simulink model "Drive_Cycle_Sim"  (R2020a)
settings: Solver=FixedStepAuto  StartTime=0  StopTime=108.92  FixedStep=0.01  MinStep=0.001  RelTol=1e-3
undefined symbols (not defined in the file or in its folder): Accumulator, Brakes, Driver, Gearbox, k_coulombToampHour, k_joulesTokWH, Motor, PedalMap, Regen, SimVehicle, Speed, Tire
libraries: autolibshared x3, simulink x2, dspstat3 x1
settings Model: Creator=Harjot  LastModifiedBy=harjo

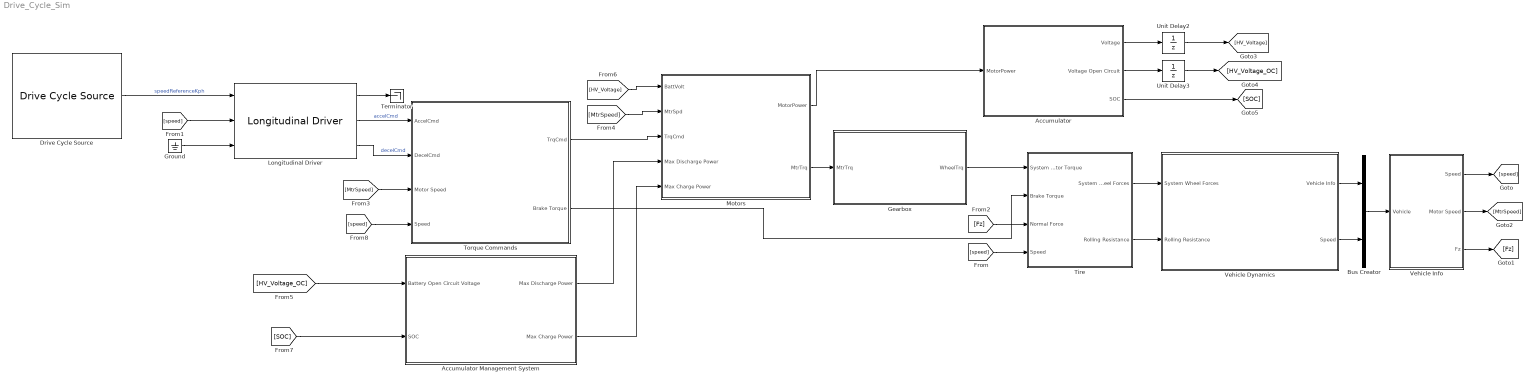
== system Drive_Cycle_Sim ==
  Accumulator : Subsystem
      mask Display: image('C:\Users\harjo\Downloads\battery.png'); % Use "Edit Image" on toolstrip to change.
  Accumulator Management System : Subsystem
      mask Display: image('C:\Users\harjo\Downloads\ams.jpg'); % Use "Edit Image" on toolstrip to change.
  Bus Creator : BusCreator  Inputs=2
  Drive Cycle Source : autolibshared/Drive Cycle Source  cycleVar=Workspace variable  wsVar=drivecycle  fileVar=cycleFTP75.mat  tfinal="108.92  seconds, Cyclic"  cycleRepeat=on  outAccPort=off  outGearPort=off  gearList=No gear data  t_wot1=5  xdot_woto=0  xdot_wot1=30  t_wot2=20  xdot_wot2=0  t_wotend=30  srcUnit=km/h  outUnit=km/hr  srcAccUnit=m/s/s  outAccUnit=m/s^2  dt=0.01  aMode=2  faultOption=off  velBnd=2  velBndUnit=mph  inUnit=m/s  timeBnd=1  failOption=off  stopSim=off  maxFaultCnt=10  maxFaultTime=2  maxTotFaultTime=15  traceOption=off  dtTrace=1  traceWindow=10  lastDCname=Custom Data Set  lastOutUnit=mph  lastDT=0.01  lastTB=1  lastSB=2  forceCalcBound=off
      settings: SourceProductBaseCode=PW,MT,VE,VP
  Gearbox : Subsystem
      mask Display: image('C:\Users\harjo\Downloads\gearbox.png'); % Use "Edit Image" on toolstrip to change.
  Ground : Ground
  Longitudinal Driver : autolibshared/Longitudinal Driver  extAccelOvr=off  extDecelOvr=off  extAccelHld=off  extDecelHld=off  extAccelZero=off  extDecelZero=off  cntrlType=PI  shftType=None  velUnits=km/hr  gearOut=off  Kp=Driver.k_kp  Ki=Driver.k_ki  Kff=Driver.k_kff  Kg=Driver.k_kg  VehVelVec=[0 100]  KffVec=[.1 .1]  KpVec=[10 10]  KiVec=[5 5]  KgVec=[0 0]  m=1500  Kpt=3000  tau=.1  L=2  aR=200  bR=2.5  cR=.5  g=9.81  vnom=Driver.k_vnom  Kaw=Driver.k_kaw  tauerr=Driver.k_tauerr  tauPt=2  GearInit=0  tShift=.1  pdlVec=[0.1 0.4 0.5 0.9]  upShftTbl=[-1 12.9375 26.4375 39.9375 51.18749999999999 62.4375 72.84375 83.25;-1 16.3125 29.8125 43.3125 54.5624 65.8125 76.78125 87.75;-1 19.6875 33.1875 46.68749999999999 57.9375 69.1875 80.71875 92.25;-1 33 52.5 77.25 100.5 138.75 161.875 185]  dwnShftTbl=[1 9.5625 23.0625 36.5625 47.8125 59.0625 68.90625 78.75;1 12.9375 26.4375 39.9375 51.18749999999999 62.4375 72.84375 83.25;1 16.3125 29.8125 43.3125 54.562499 65.8125 76.78125 87.75;1 19.6875 33.1875 46.68749999999999 57.9375 69.1875 80.71875 92.25]  tClutch=.5  tRev=.5  tPark=120  aMode=1  UpGearVec="[0  1  2  3  4  5  6  7]"  DownGearVec="[1  2  3  4  5  6  7  8]"
      settings: SourceProductBaseCode=PW,MT,VE,VP
  Motors : Subsystem
      mask Display: image('C:\Users\harjo\Downloads\motor.png'); % Use "Edit Image" on toolstrip to change.
  Terminator : Terminator
  Tire : Subsystem
      mask Display: image('C:\Users\harjo\Downloads\tire.jpg'); % Use "Edit Image" on toolstrip to change.
  Torque Commands : Subsystem
  Unit Delay2 : UnitDelay  InitialCondition=Accumulator.k_initialPackVoltage  SampleTime=-1  HasFrameUpgradeWarning=on
  Unit Delay3 : UnitDelay  InitialCondition=Accumulator.k_maxCellVoltage  SampleTime=-1  HasFrameUpgradeWarning=on
  Vehicle Dynamics : Subsystem
      mask Display: image('C:\Users\harjo\Downloads\carZapdos.png'); % Use "Edit Image" on toolstrip to change.
  Vehicle Info : Subsystem
  wires:
  Gearbox/1(WheelTrq) -> Tire/1(System Motor Torque)
  [MtrSpeed] -> Torque Commands/3(Motor Speed)
  Torque Commands/2(Brake Torque) -> Tire/2(Brake Torque)
  Tire/2(Rolling Resistance) -> Vehicle Dynamics/2(Rolling Resistance)
  Tire/1(System Wheel Forces) -> Vehicle Dynamics/1(System Wheel Forces)
  Drive Cycle Source/1 -> Longitudinal Driver/1  "speedReferenceKph"
  [Fz] -> Tire/3(Normal Force)
  [speed] -> Tire/4(Speed)
  Unit Delay2/1 -> [HV_Voltage]
  Accumulator/1(Voltage) -> Unit Delay2/1
  [HV_Voltage] -> Motors/1(BattVolt)
  Accumulator/2(Voltage Open Circuit) -> Unit Delay3/1
  Unit Delay3/1 -> [HV_Voltage_OC]
  [MtrSpeed] -> Motors/2(MtrSpd)
  Motors/1(MotorPower) -> Accumulator/1(MotorPower)
  Motors/2(MtrTrq) -> Gearbox/1(MtrTrq)
  Torque Commands/1(TrqCmd) -> Motors/3(TrqCmd)
  [HV_Voltage_OC] -> Accumulator Management System/1(Battery Open Circuit Voltage)
  Accumulator Management System/1(Max Discharge Power) -> Motors/4(Max Discharge Power)
  [speed] -> Longitudinal Driver/2
  Longitudinal Driver/1 -> Terminator/1
  Longitudinal Driver/3 -> Torque Commands/2(DecelCmd)  "decelCmd"
  Longitudinal Driver/2 -> Torque Commands/1(AccelCmd)  "accelCmd"
  Ground/1 -> Longitudinal Driver/3
  Vehicle Dynamics/1(Vehicle Info) -> Bus Creator/1
  Vehicle Dynamics/2(Speed) -> Bus Creator/2
  Bus Creator/1 -> Vehicle Info/1(Vehicle)
  Vehicle Info/1(Speed) -> [speed]
  Vehicle Info/3(Fz) -> [Fz]
  Vehicle Info/2(Motor Speed) -> [MtrSpeed]
  Accumulator/3(SOC) -> [SOC]
  [SOC] -> Accumulator Management System/2(SOC)
  Accumulator Management System/2(Max Charge Power) -> Motors/5(Max Charge Power)
  [speed] -> Torque Commands/4(Speed)

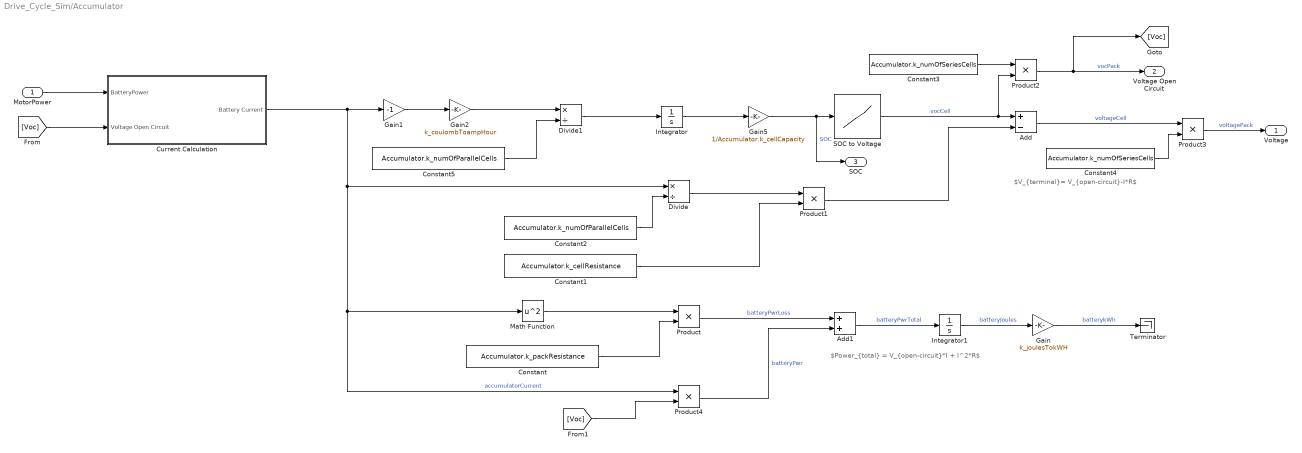
== system Drive_Cycle_Sim/Accumulator ==
  note: $V_{terminal}= V_{open-circuit}-I*R$
  note: $Power_{total} = V_{open-circuit}*I + I^2*R$
  MotorPower : Inport  Unit=W
  Add : Sum  Inputs=+-
  Add1 : Sum
  Constant : Constant  Value=Accumulator.k_packResistance
  Constant1 : Constant  Value=Accumulator.k_cellResistance
  Constant2 : Constant  Value=Accumulator.k_numOfParallelCells
  Constant3 : Constant  Value=Accumulator.k_numOfSeriesCells
  Constant4 : Constant  Value=Accumulator.k_numOfSeriesCells
  Constant5 : Constant  Value=Accumulator.k_numOfParallelCells
  Current Calculation : Subsystem
  Divide : Product  Inputs=*/
  Divide1 : Product  Inputs=*/
  Gain : Gain  Gain=k_joulesTokWH
  Gain1 : Gain  Gain=-1
  Gain2 : Gain  Gain=k_coulombToampHour
  Gain5 : Gain  Gain=1/Accumulator.k_cellCapacity
  Integrator : Integrator  InitialCondition=Accumulator.k_initialCellCapacity
  Integrator1 : Integrator  InitialCondition=Accumulator.k_packCapacity
  Math Function : Math  Operator=square  SaturateOnIntegerOverflow=on
  Product{,1..4} (5 alike) : Product  RndMeth=Zero
  SOC to Voltage : Lookup_n-D  NumberOfTableDimensions=1  BreakpointsForDimension1=Accumulator.k_cellSOCBreakPoints  Table=Accumulator.k_cellOpenVoltageLookupTable  ExtrapMethod=Clip  InternalRulePriority=Speed  RndMeth=Simplest  InputSameDT=on
  Terminator : Terminator
  Voltage : Outport  Unit=V
  Voltage Open Circuit : Outport  Port=2  Unit=V
  SOC : Outport  Port=3
  wires:
  Add/1 -> Product3/1  "voltageCell"
  Integrator/1 -> Gain5/1
  Product/1 -> Add1/1  "batteryPwrLoss"
  Product1/1 -> Add/2
  SOC to Voltage/1 -> Product2/2, Add/1  "vocCell"
  Product3/1 -> Voltage/1  "voltagePack"
  Gain5/1 -> SOC/1, SOC to Voltage/1  "SOC"
  MotorPower/1 -> Current Calculation/1(BatteryPower)
  Product2/1 -> [Voc], Voltage Open Circuit/1  "vocPack"
  [Voc] -> Current Calculation/2(Voltage Open Circuit)
  Current Calculation/1(Battery Current) -> Gain1/1, Divide/1, Math Function/1, Product4/1  "accumulatorCurrent"
  Math Function/1 -> Product/1
  Constant/1 -> Product/2
  Constant1/1 -> Product1/2
  Divide/1 -> Product1/1
  Constant2/1 -> Divide/2
  Constant3/1 -> Product2/1
  Constant4/1 -> Product3/2
  Product4/1 -> Add1/2  "batteryPwr"
  [Voc] -> Product4/2
  Add1/1 -> Integrator1/1  "batteryPwrTotal"
  Divide1/1 -> Integrator/1
  Integrator1/1 -> Gain/1  "batteryJoules"
  Gain/1 -> Terminator/1  "batterykWh"
  Gain1/1 -> Gain2/1
  Constant5/1 -> Divide1/2
  Gain2/1 -> Divide1/1

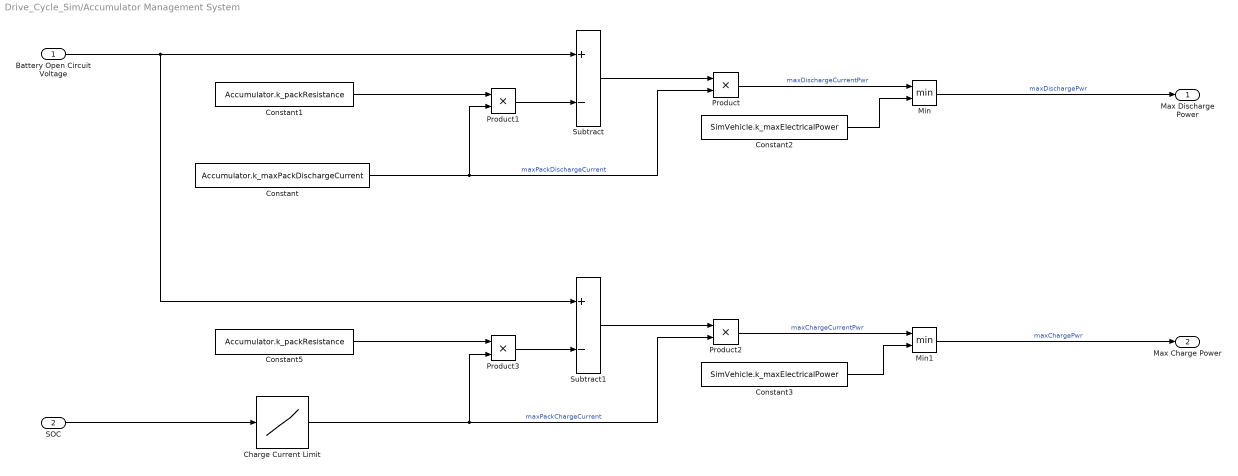
== system Drive_Cycle_Sim/Accumulator Management System ==
  Battery Open Circuit Voltage : Inport  Unit=V
  SOC : Inport  Port=2
  Charge Current Limit : Lookup_n-D  NumberOfTableDimensions=1  BreakpointsForDimension1=Accumulator.k_chargeLimitSOCBreakPoints  Table=Accumulator.k_chargeLimitLookuptable  ExtrapMethod=Clip  InternalRulePriority=Speed  RndMeth=Simplest  InputSameDT=on
  Constant : Constant  Value=Accumulator.k_maxPackDischargeCurrent
  Constant1 : Constant  Value=Accumulator.k_packResistance
  Constant2 : Constant  Value=SimVehicle.k_maxElectricalPower
  Constant3 : Constant  Value=SimVehicle.k_maxElectricalPower
  Constant5 : Constant  Value=Accumulator.k_packResistance
  Min : MinMax  Inputs=2
  Min1 : MinMax  Inputs=2
  Product{,1..3} (4 alike) : Product
  Subtract : Sum  Inputs=+-
  Subtract1 : Sum  Inputs=+-
  Max Discharge Power : Outport  Unit=W
  Max Charge Power : Outport  Port=2  Unit=W
  wires:
  Constant/1 -> Product/2, Product1/2  "maxPackDischargeCurrent"
  Subtract/1 -> Product/1
  Product/1 -> Min/1  "maxDischargeCurrentPwr"
  Constant1/1 -> Product1/1
  Product1/1 -> Subtract/2
  Min/1 -> Max Discharge Power/1  "maxDischargePwr"
  Constant2/1 -> Min/2
  Min1/1 -> Max Charge Power/1  "maxChargePwr"
  Product2/1 -> Min1/1  "maxChargeCurrentPwr"
  Subtract1/1 -> Product2/1
  Constant3/1 -> Min1/2
  Battery Open Circuit Voltage/1 -> Subtract1/1, Subtract/1
  Charge Current Limit/1 -> Product3/2, Product2/2  "maxPackChargeCurrent"
  Constant5/1 -> Product3/1
  Product3/1 -> Subtract1/2
  SOC/1 -> Charge Current Limit/1

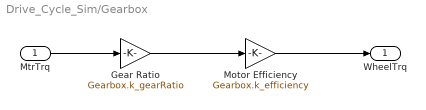
== system Drive_Cycle_Sim/Gearbox ==
  MtrTrq : Inport  Unit=N*m
  Gear Ratio : Gain  Gain=Gearbox.k_gearRatio
  Motor Efficiency : Gain  Gain=Gearbox.k_efficiency
  WheelTrq : Outport  Unit=N*m
  wires:
  Gear Ratio/1 -> Motor Efficiency/1
  MtrTrq/1 -> Gear Ratio/1
  Motor Efficiency/1 -> WheelTrq/1

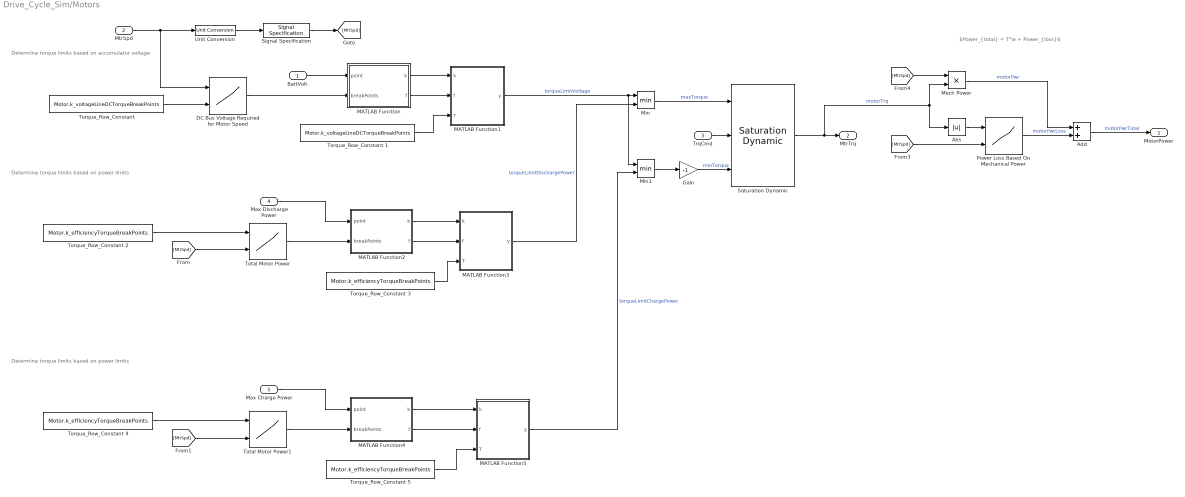
== system Drive_Cycle_Sim/Motors ==
  note: Determine torque limits based on accumulator voltage
  note: Determine torque limits based on power limits
  note: $Power_{total} = T*w + Power_{loss}$
  note: Determine torque limits based on power limits
  BattVolt : Inport  Unit=V
  MtrSpd : Inport  Port=2  Unit=rpm
  TrqCmd : Inport  Port=3  Unit=N*m
  Max Discharge Power : Inport  Port=4  Unit=W
  Max Charge Power : Inport  Port=5  Unit=W
  Abs : Abs
  Add : Sum
  DC Bus Voltage Required for Motor Speed : Lookup_n-D  BreakpointsForDimension1=Speed(:,1)  BreakpointsForDimension2=Motor.k_voltageLineDCTorqueBreakPoints  Table=Motor.k_voltageLineDCLookpupTable  InternalRulePriority=Speed  OutDataTypeStr=double  RndMeth=Simplest  InputSameDT=on
  Gain : Gain  Gain=-1
  MATLAB Function : MATLAB Function  TreatAsAtomicUnit=on
  MATLAB Function1 : MATLAB Function  TreatAsAtomicUnit=on
  MATLAB Function2 : MATLAB Function  TreatAsAtomicUnit=on
  MATLAB Function3 : MATLAB Function  TreatAsAtomicUnit=on
  MATLAB Function4 : MATLAB Function  TreatAsAtomicUnit=on
  MATLAB Function5 : MATLAB Function  TreatAsAtomicUnit=on
  Mech Power : Product
  Min : MinMax  Inputs=2
  Min1 : MinMax  Inputs=2
  Power Loss Based On Mechanical Power : Lookup_n-D  BreakpointsForDimension1=Motor.k_efficiencyTorqueBreakPoints  BreakpointsForDimension2=Motor.k_efficiencyMotorSpeedBreakPoints  Table=Motor.k_powerLossLookupTable  InternalRulePriority=Speed  RndMeth=Simplest  InputSameDT=on
  Saturation Dynamic : simulink/Discontinuities/Saturation Dynamic  OutMin=[]  OutMax=[]  OutDataTypeStr=Inherit: Same as second input  OutDataType=fixdt(1, 16)  OutScaling=2^-10  DoSatur=off
  Signal Specification : SignalSpecification  Unit=rad/s
  "Torque_Row_Constant " : Constant  Value=Motor.k_voltageLineDCTorqueBreakPoints
  Torque_Row_Constant 1 : Constant  Value=Motor.k_voltageLineDCTorqueBreakPoints
  Torque_Row_Constant {2..5} (4 alike) : Constant  Value=Motor.k_efficiencyTorqueBreakPoints
  Total Motor Power : Lookup_n-D  BreakpointsForDimension1=Motor.k_efficiencyTorqueBreakPoints  BreakpointsForDimension2=Motor.k_efficiencyMotorSpeedBreakPoints  Table=Motor.k_totalDischargeMotorPowerLookupTable  InternalRulePriority=Speed  RndMeth=Simplest  InputSameDT=on
  Total Motor Power1 : Lookup_n-D  BreakpointsForDimension1=Motor.k_efficiencyTorqueBreakPoints  BreakpointsForDimension2=Motor.k_efficiencyMotorSpeedBreakPoints  Table=Motor.k_totalChargeMotorPowerLookupTable  InternalRulePriority=Speed  RndMeth=Simplest  InputSameDT=on
  Unit Conversion : UnitConversion
  MotorPower : Outport
  MtrTrq : Outport  Port=2
  wires:
  Power Loss Based On Mechanical Power/1 -> Add/2  "motorPwrLoss"
  Mech Power/1 -> Add/1  "motorPwr"
  MATLAB Function/1(k) -> MATLAB Function1/1(k)
  TrqCmd/1 -> Saturation Dynamic/2
  MATLAB Function/2(f) -> MATLAB Function1/2(f)
  "Torque_Row_Constant "/1 -> DC Bus Voltage Required for Motor Speed/2
  Saturation Dynamic/1 -> Abs/1, Mech Power/2, MtrTrq/1  "motorTrq"
  MtrSpd/1 -> DC Bus Voltage Required for Motor Speed/1, Unit Conversion/1
  BattVolt/1 -> MATLAB Function/1(point)
  DC Bus Voltage Required for Motor Speed/1 -> MATLAB Function/2(breakPoints)
  Torque_Row_Constant 1/1 -> MATLAB Function1/3(T)
  Unit Conversion/1 -> Signal Specification/1
  Signal Specification/1 -> [MtrSpd]
  Max Discharge Power/1 -> MATLAB Function2/1(point)
  Total Motor Power/1 -> MATLAB Function2/2(breakPoints)
  MATLAB Function2/1(k) -> MATLAB Function3/1(k)
  MATLAB Function2/2(f) -> MATLAB Function3/2(f)
  Torque_Row_Constant 3/1 -> MATLAB Function3/3(T)
  MATLAB Function1/1(y) -> Min1/1, Min/1  "torqueLimitVoltage"
  MATLAB Function3/1(y) -> Min/2  "torqueLimitDischargePower"
  Min/1 -> Saturation Dynamic/1  "maxTorque"
  [MtrSpd] -> Total Motor Power/2
  Torque_Row_Constant 2/1 -> Total Motor Power/1
  Add/1 -> MotorPower/1  "motorPwrTotal"
  [MtrSpd] -> Power Loss Based On Mechanical Power/2
  [MtrSpd] -> Mech Power/1
  Torque_Row_Constant 4/1 -> Total Motor Power1/1
  MATLAB Function4/2(f) -> MATLAB Function5/2(f)
  MATLAB Function4/1(k) -> MATLAB Function5/1(k)
  Torque_Row_Constant 5/1 -> MATLAB Function5/3(T)
  [MtrSpd] -> Total Motor Power1/2
  Total Motor Power1/1 -> MATLAB Function4/2(breakPoints)
  Max Charge Power/1 -> MATLAB Function4/1(point)
  Min1/1 -> Gain/1
  MATLAB Function5/1(y) -> Min1/2  "torqueLimitChargePower"
  Gain/1 -> Saturation Dynamic/3  "minTorque"
  Abs/1 -> Power Loss Based On Mechanical Power/1

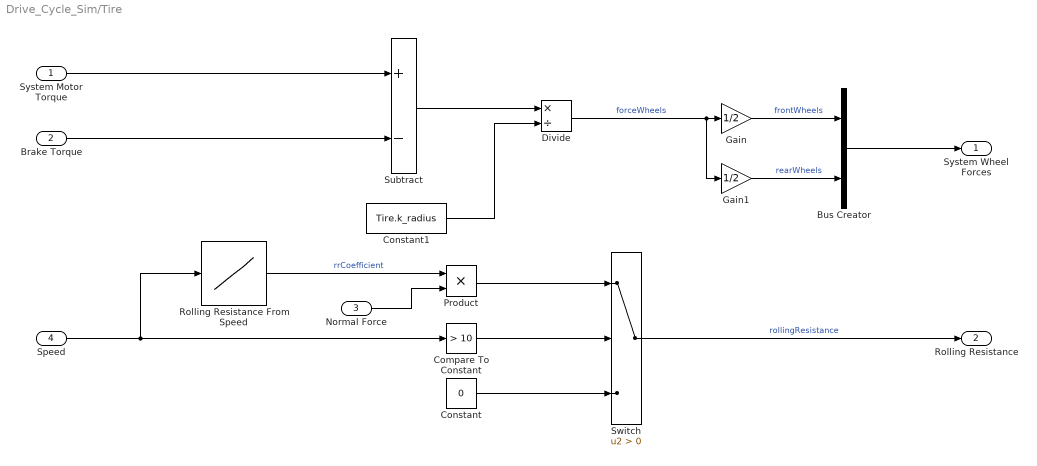
== system Drive_Cycle_Sim/Tire ==
  System Motor Torque : Inport  Unit=N*m
  Brake Torque : Inport  Port=2  Unit=N*m
  Normal Force : Inport  Port=3  Unit=N
  Speed : Inport  Port=4  Unit=km/hr
  Bus Creator : BusCreator  Inputs=2
  Compare To Constant : simulink/Logic and Bit Operations/Compare To Constant  relop=>  const=10  OutDataTypeStr=boolean
  Constant : Constant  Value=0
  Constant1 : Constant  Value=Tire.k_radius
  Divide : Product  Inputs=*/
  Gain : Gain  Gain=1/2
  Gain1 : Gain  Gain=1/2
  Product : Product
  Rolling Resistance From Speed : Lookup_n-D  NumberOfTableDimensions=1  BreakpointsForDimension1=Tire.k_rollingRadiusSpeedBreakPoints  Table=Tire.k_rollingRadiusLookup  ExtrapMethod=Clip  InternalRulePriority=Speed  RndMeth=Simplest  InputSameDT=on
  Subtract : Sum  Inputs=+-
  Switch : Switch  Criteria=u2 > Threshold
  System Wheel Forces : Outport  Unit=N
  Rolling Resistance : Outport  Port=2  Unit=N
  wires:
  Brake Torque/1 -> Subtract/2
  Bus Creator/1 -> System Wheel Forces/1
  System Motor Torque/1 -> Subtract/1
  Gain/1 -> Bus Creator/1  "frontWheels"
  Gain1/1 -> Bus Creator/2  "rearWheels"
  Compare To Constant/1 -> Switch/2
  Speed/1 -> Rolling Resistance From Speed/1, Compare To Constant/1
  Constant/1 -> Switch/3
  Product/1 -> Switch/1
  Switch/1 -> Rolling Resistance/1  "rollingResistance"
  Normal Force/1 -> Product/2
  Rolling Resistance From Speed/1 -> Product/1  "rrCoefficient"
  Subtract/1 -> Divide/1
  Constant1/1 -> Divide/2
  Divide/1 -> Gain1/1, Gain/1  "forceWheels"

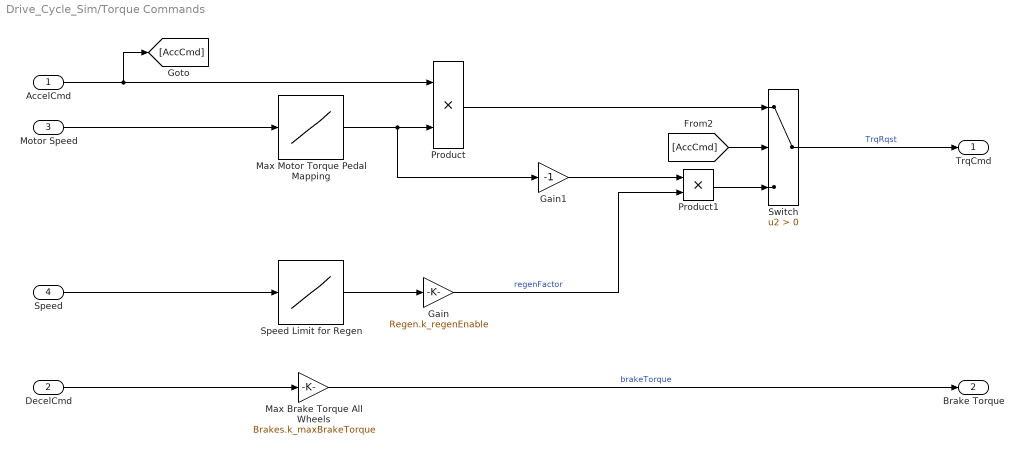
== system Drive_Cycle_Sim/Torque Commands ==
  AccelCmd : Inport
  DecelCmd : Inport  Port=2
  Motor Speed : Inport  Port=3  Unit=rpm
  Speed : Inport  Port=4  Unit=km/hr
  Gain : Gain  Gain=Regen.k_regenEnable
  Gain1 : Gain  Gain=-1
  Max Brake Torque All Wheels : Gain  Gain=Brakes.k_maxBrakeTorque
  Max Motor Torque Pedal Mapping : Lookup_n-D  NumberOfTableDimensions=1  BreakpointsForDimension1=PedalMap.k_motorRPMBreakPoints  Table=PedalMap.k_maxTorqueLookupTable  ExtrapMethod=Clip  InternalRulePriority=Speed  RndMeth=Simplest  InputSameDT=on
  Product : Product
  Product1 : Product
  Speed Limit for Regen : Lookup_n-D  NumberOfTableDimensions=1  BreakpointsForDimension1=Regen.k_regenFactorSpeedBreakPoints  Table=Regen.k_regenFactorSpeedLookupTable  ExtrapMethod=Clip  InternalRulePriority=Speed  RndMeth=Simplest  InputSameDT=on
  Switch : Switch  Criteria=u2 > Threshold
  TrqCmd : Outport  Unit=N*m
  Brake Torque : Outport  Port=2  Unit=N*m
  wires:
  AccelCmd/1 -> [AccCmd], Product/1
  Motor Speed/1 -> Max Motor Torque Pedal Mapping/1
  Max Motor Torque Pedal Mapping/1 -> Gain1/1, Product/2
  Max Brake Torque All Wheels/1 -> Brake Torque/1  "brakeTorque"
  [AccCmd] -> Switch/2
  Switch/1 -> TrqCmd/1  "TrqRqst"
  Speed Limit for Regen/1 -> Gain/1
  Product1/1 -> Switch/3
  Product/1 -> Switch/1
  Gain/1 -> Product1/2  "regenFactor"
  Gain1/1 -> Product1/1
  DecelCmd/1 -> Max Brake Torque All Wheels/1
  Speed/1 -> Speed Limit for Regen/1

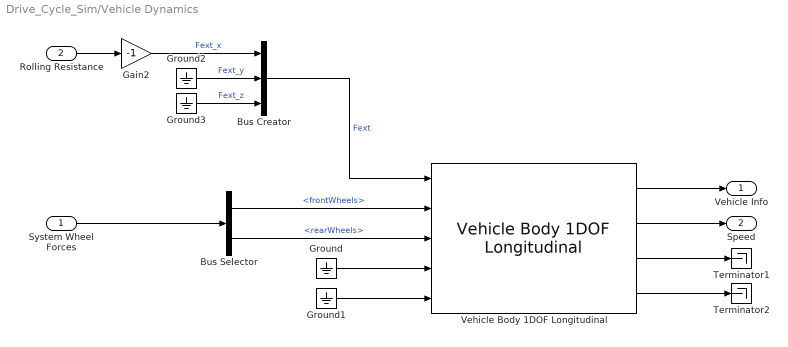
== system Drive_Cycle_Sim/Vehicle Dynamics ==
  System Wheel Forces : Inport  Unit=N
  Rolling Resistance : Inport  Port=2  Unit=N
  Bus Creator : BusCreator  Inputs=3
  Bus Selector : BusSelector  OutputSignals=frontWheels,rearWheels
  Gain2 : Gain  Gain=-1
  Ground{,1..3} (4 alike) : Ground
  Terminator1 : Terminator
  Terminator2 : Terminator
  Vehicle Body 1DOF Longitudinal : autolibshared/Vehicle Body 1DOF Longitudinal  VariantControl=SL  extFMode=on  extMMode=off  extTamb=off  wind3D=off  aMode=1  NF=2  NR=2  m=SimVehicle.k_totalMass  a=SimVehicle.k_distanceCOMtoFrontAxle  b=SimVehicle.k_distanceCOMtoRearAxle  h=SimVehicle.k_heightOfCenterOfMass  Cd=SimVehicle.k_dragCoefficient  Cl=0  Cpm=0  Af=SimVehicle.k_frontArea  x_o=0  xdot_o=0  Pabs=101325  T=273  g=9.81
      settings: SourceProductBaseCode=PW,MT,VE,VP
  Vehicle Info : Outport
  Speed : Outport  Port=2  Unit=m/s
  wires:
  Rolling Resistance/1 -> Gain2/1
  Vehicle Body 1DOF Longitudinal/1 -> Vehicle Info/1
  Vehicle Body 1DOF Longitudinal/3 -> Terminator1/1
  Vehicle Body 1DOF Longitudinal/4 -> Terminator2/1
  Vehicle Body 1DOF Longitudinal/2 -> Speed/1
  Gain2/1 -> Bus Creator/1  "Fext_x"
  Ground2/1 -> Bus Creator/2  "Fext_y"
  Ground3/1 -> Bus Creator/3  "Fext_z"
  System Wheel Forces/1 -> Bus Selector/1
  Bus Creator/1 -> Vehicle Body 1DOF Longitudinal/1  "Fext"
  Ground/1 -> Vehicle Body 1DOF Longitudinal/4
  Ground1/1 -> Vehicle Body 1DOF Longitudinal/5
  Bus Selector/1 -> Vehicle Body 1DOF Longitudinal/2  "<frontWheels>"
  Bus Selector/2 -> Vehicle Body 1DOF Longitudinal/3  "<rearWheels>"

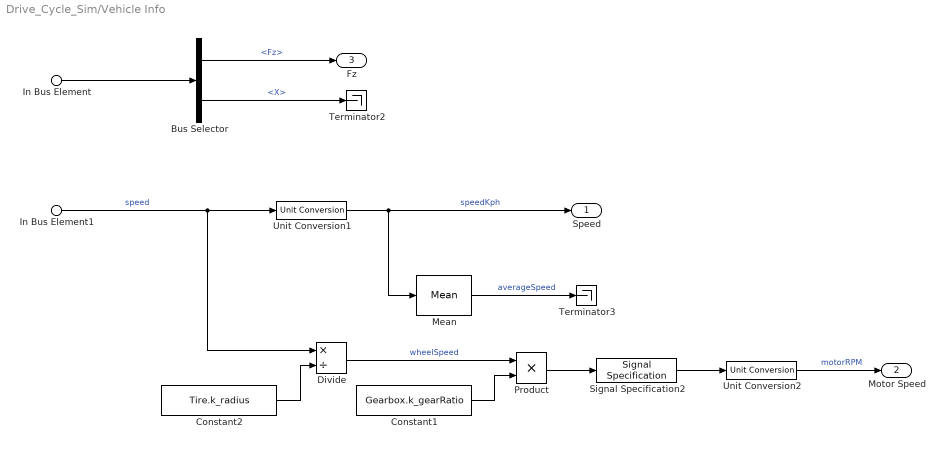
== system Drive_Cycle_Sim/Vehicle Info ==
  In Bus Element : Inport  PortName=Vehicle  Element=Info
  In Bus Element1 : Inport  PortName=Vehicle  Element=xdot
  Bus Selector : BusSelector  OutputSignals=BdyFrm.Forces.Grvty.Fz,InertFrm.Cg.Disp.X
  Constant1 : Constant  Value=Gearbox.k_gearRatio
  Constant2 : Constant  Value=Tire.k_radius
  Divide : Product  Inputs=*/
  Mean : dspstat3/Mean  run=on  InputProcessing=Columns as channels (frame based)  reset_popup=None  directionMode=Each column  dimension=1  roiEnable=off  roiType=Rectangles  roiPortion=Entire ROI  roiOutput=Individual statistics for each ROI  roiFlag=off  roundingMode=Floor  overflowMode=off  outputDataTypeStr=Inherit: Same as accumulator  outputMin=[]  outputMax=[]  outputLastDataTypeStr=Inherit: Same as accumulator
  Product : Product
  Signal Specification2 : SignalSpecification  Unit=rad/s
  Terminator2 : Terminator
  Terminator3 : Terminator
  Unit Conversion1 : UnitConversion
  Unit Conversion2 : UnitConversion
  Speed : Outport  Unit=km/hr
  Motor Speed : Outport  Port=2  Unit=rpm
  Fz : Outport  Port=3  Unit=N
  wires:
  Unit Conversion1/1 -> Mean/1, Speed/1  "speedKph"
  Signal Specification2/1 -> Unit Conversion2/1
  Bus Selector/1 -> Fz/1  "<Fz>"
  Constant2/1 -> Divide/2
  In Bus Element1/1 -> Divide/1, Unit Conversion1/1  "speed"
  In Bus Element/1 -> Bus Selector/1
  Bus Selector/2 -> Terminator2/1  "<X>"
  Unit Conversion2/1 -> Motor Speed/1  "motorRPM"
  Product/1 -> Signal Specification2/1
  Divide/1 -> Product/1  "wheelSpeed"
  Constant1/1 -> Product/2
  Mean/1 -> Terminator3/1  "averageSpeed"

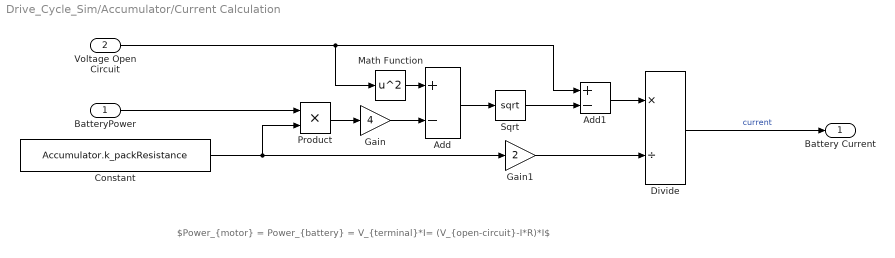
== system Drive_Cycle_Sim/Accumulator/Current Calculation ==
  note: $Power_{motor} = Power_{battery} = V_{terminal}*I= (V_{open-circuit}-I*R)*I$
  BatteryPower : Inport
  Voltage Open Circuit : Inport  Port=2
  Add : Sum  Inputs=+-
  Add1 : Sum  Inputs=+-
  Constant : Constant  Value=Accumulator.k_packResistance
  Divide : Product  Inputs=*/
  Gain : Gain  Gain=4
  Gain1 : Gain  Gain=2
  Math Function : Math  Operator=square  SignedPower=on  SaturateOnIntegerOverflow=on
  Product : Product  RndMeth=Zero
  Sqrt : Sqrt  SaturateOnIntegerOverflow=on
  Battery Current : Outport  Unit=A  VectorParamsAs1DForOutWhenUnconnected=off
  wires:
  BatteryPower/1 -> Product/1
  Constant/1 -> Gain1/1, Product/2
  Product/1 -> Gain/1
  Voltage Open Circuit/1 -> Math Function/1, Add1/1
  Math Function/1 -> Add/1
  Gain/1 -> Add/2
  Sqrt/1 -> Add1/2
  Add/1 -> Sqrt/1
  Add1/1 -> Divide/1
  Gain1/1 -> Divide/2
  Divide/1 -> Battery Current/1  "current"

== matlab function Drive_Cycle_Sim/Motors/MATLAB Function1 ==
  data: k input; y output; f input; T input
function y = fcn(k,f,T)
if(f == 0)
    y = T(k);
else
    diff = T(k+1) - T(k);
    y = T(k) + f*diff;
end

== matlab function Drive_Cycle_Sim/Motors/MATLAB Function ==
  data: point input; k output; breakPoints input; f output
function [k,f] = fcn(point,breakPoints)
if(point >= breakPoints)
    k = length(breakPoints);
    f = 0;
    return
elseif(point <= breakPoints)
    k = 1;
    f = 0;
else
    endIndex = length(breakPoints);
    for i = 1:length(breakPoints)
        if(point <= breakPoints(i))
            endIndex = i;
        break
        end
    end
    k = endIndex - 1;
    f = (point - breakPoints(k))/(breakPoints(endIndex) - breakPoints(k));
end

== matlab function Drive_Cycle_Sim/Motors/MATLAB Function2 ==
  data: point input; k output; breakPoints input; f output
function [k,f] = fcn(point,breakPoints)
if(point >= breakPoints)
    k = length(breakPoints);
    f = 0;
    return
elseif(point <= breakPoints)
    k = 1;
    f = 0;
else
    endIndex = length(breakPoints);
    for i = 1:length(breakPoints)
        if(point <= breakPoints(i))
            endIndex = i;
        break
        end
    end
    k = endIndex - 1;
    f = (point - breakPoints(k))/(breakPoints(endIndex) - breakPoints(k));
end

== matlab function Drive_Cycle_Sim/Motors/MATLAB Function3 ==
  data: k input; y output; f input; T input
function y = fcn(k,f,T)
if(f == 0)
    y = T(k);
else
    diff = T(k+1) - T(k);
    y = T(k) + f*diff;
end

== matlab function Drive_Cycle_Sim/Motors/MATLAB Function4 ==
  data: point input; k output; breakPoints input; f output
function [k,f] = fcn(point,breakPoints)
if(point >= breakPoints)
    k = length(breakPoints);
    f = 0;
    return
elseif(point <= breakPoints)
    k = 1;
    f = 0;
else
    endIndex = length(breakPoints);
    for i = 1:length(breakPoints)
        if(point <= breakPoints(i))
            endIndex = i;
        break
        end
    end
    k = endIndex - 1;
    f = (point - breakPoints(k))/(breakPoints(endIndex) - breakPoints(k));
end

== matlab function Drive_Cycle_Sim/Motors/MATLAB Function5 ==
  data: k input; y output; f input; T input
function y = fcn(k,f,T)
if(f == 0)
    y = T(k);
else
    diff = T(k+1) - T(k);
    y = T(k) + f*diff;
end
